simulink model "sfediticon"  (Simulink 7.6)
settings: Solver=FixedStepDiscrete  StartTime=0.0  StopTime=inf  RelTol=1e-3
CloseFcn:
  | sf_edit_icon('kill');
settings Model: Creator=The MathWorks Inc.  CovMetricSettings=dcmtr  ExtModeTrigMode=oneshot  ExtModeArmWhenConnect=off  ExtModeAutoUpdateStatusClock=off
settings DataIOCC: LimitDataPoints=off  SaveOutput=off  SaveTime=off
settings OptimizationCC: BooleanDataType=off  InlineInvariantSignals=on  InitFltsAndDblsToZero=on  EfficientMapNaN2IntZero=off
settings DebuggingCC: SaveWithParameterizedLinksMsg=none  SignalResolutionControl=TryResolveAllWithWarning  SolverPrmCheckMsg=none  MultiTaskDSMMsg=warning  MultiTaskCondExecSysMsg=none  StrictBusMsg=None
settings HardwareCC: TargetUnknown=on
settings SFSimCC: SimCustomHeaderCode=#define IS_MEX_TARGET 0  SimParseCustomCode=off
settings RTWCC: IncludeERTFirstTime=on
settings GRTTargetCC: TargetFcnLib=ansi_tfl_tmw.mat

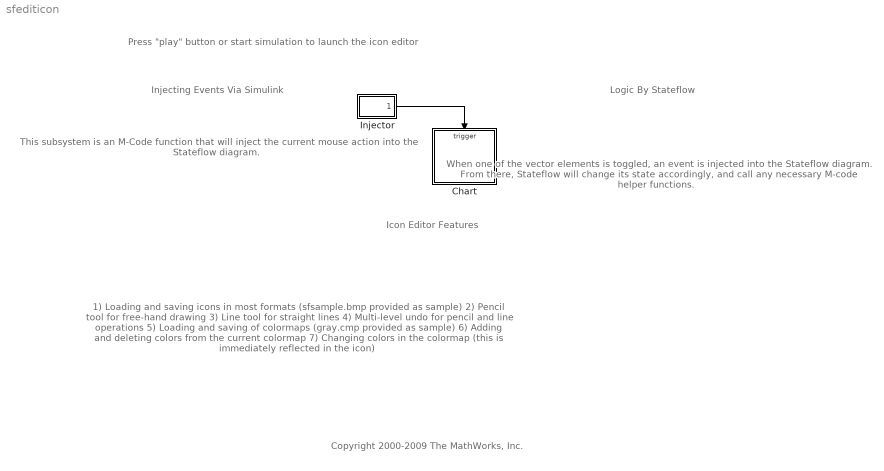
== system sfediticon ==
  note: This subsystem is an M-Code
      | function that will inject the
      | current mouse action into the
      | Stateflow diagram.
  note: Injecting Events
      | Via Simulink
  note: When one of the vector elements
      | is toggled, an event is injected
      | into the Stateflow diagram.
      | From there, Stateflow will
      | change its state accordingly,
      | and call any necessary M-code
      | helper functions.
  note: Logic By Stateflow
  note: 1) Loading and saving icons in most formats
      |      (sfsample.bmp provided as sample)
      | 2) Pencil tool for free-hand drawing
      | 3) Line tool for straight lines
      | 4) Multi-level undo for pencil and line operations
      | 5) Loading and saving of colormaps
      |      (gray.cmp provided as sample)
      | 6) Adding and deleting colors from the current
      |      colormap
      | 7) Changing colors in the colormap
      |     (this is immediately reflected in the icon)
  note: Icon Editor Features
  note: Press "play" button or start simulation to launch the icon editor
  note: Copyright 2000-2009 The MathWorks, Inc.
  Chart : Stateflow chart  TreatAsAtomicUnit=on
  Injector : Subsystem
  wires:
  Injector/1(Event) -> Chart/Trigger

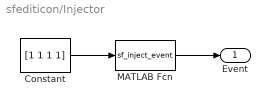
== system sfediticon/Injector ==
  Constant : Constant  Value=[1 1 1 1]
  MATLAB Fcn : MATLABFcn  MATLABFcn=sf_inject_event
  Event : Outport
  wires:
  MATLAB Fcn/1 -> Event/1
  Constant/1 -> MATLAB Fcn/1

== stateflow chart Chart ==
  settings: executeAtInitialization=1
  state ToolBar [parallel]
    settings: executionOrder=3
    state Released
    state Locked
      en:
      ml.sf_edit_icon...
      ('status', 'Tool locked');
    state Pressed
      en:
      pressedIcon = focusedIcon;
      press(pressedIcon,1);
      ex: press(pressedIcon,0);
    state icon_operation(icon) [function]
      (default) -> (junction 26)
      (junction 26) -> (junction 27) [order 2]
      (junction 26) -> (junction 28) [order 1] : [icon == OPEN_ICON] {ml.sf_edit_icon('open');}
      (junction 33) -> (junction 32) [order 1] : [icon == SAVE_MAP_ICON] {ml.sf_edit_icon('save_map');}
      (junction 27) -> (junction 29) [order 1] : [icon == SAVE_ICON] {ml.sf_edit_icon('save_as');}
      (junction 27) -> (junction 30) [order 2]
      (junction 30) -> (junction 31) [order 1] : [icon == OPEN_MAP_ICON] {ml.sf_edit_icon('open_map');}
      (junction 33) -> (junction 34) [order 2]
      (junction 34) -> (junction 70) : [icon == UNDO_ICON] {ml.sf_edit_icon('undo');}
      (junction 30) -> (junction 33) [order 2]
    state None
      pressedIcon = 0;
      ml.sf_edit_icon('status', 'Select a tool');
      ml.sf_edit_icon('normal_cursor');
    state press(icon,sp) [function]
      (junction 42) -> (junction 25) [order 2]
      (junction 35) -> (junction 37) [order 1] : [icon == OPEN_MAP_ICON] {ml.sf_edit_icon('press',sp,'open_map');}
      (junction 38) -> (junction 44) [order 1] : [icon == SAVE_MAP_ICON] {ml.sf_edit_icon('press', sp, 'save_map');}
      (junction 40) -> (junction 36) [order 1] : [icon == SAVE_ICON] {ml.sf_edit_icon('press', sp, 'save_as');}
      (junction 40) -> (junction 35) [order 2]
      (junction 35) -> (junction 38) [order 2]
      (junction 46) -> (junction 43) [order 1] : [icon == UNDO_ICON] {ml.sf_edit_icon('press',sp,'undo');}
      (junction 42) -> (junction 58) [order 1] : [icon == LINE_ICON] {ml.sf_edit_icon('press',sp,'line');}
      (junction 46) -> (junction 42) [order 2]
      (junction 38) -> (junction 46) [order 2]
      (junction 61) -> (junction 40) [order 2]
      (default) -> (junction 61)
      (junction 61) -> (junction 39) [order 1] : [icon == OPEN_ICON] {ml.sf_edit_icon('press', sp, 'open');}
      (junction 25) -> (junction 69) : [icon == PENCIL_ICON] {ml.sf_edit_icon('press',sp,'pencil');}
    ToolBar.None -> Pressed : NBD [in(Focus.Toolbar)]
    Released -> Pressed [order 1] : BM [pressedIcon == focusedIcon]
    Pressed -> Released [order 1] : BM [pressedIcon != focusedIcon]
    (junction 62) -> ToolBar.None [order 3] : {icon_operation(pressedIcon);}
    Released -> ToolBar.None [order 2] : BU
    (junction 62) -> Locked [order 1] : [(pressedIcon == LINE_ICON)]...
        | {ml.sf_edit_icon('line_cursor');}
    Locked -> Pressed : NBD[in(Focus.Toolbar)]
    (default) -> ToolBar.None
    (junction 62) -> Locked [order 2] : [(pressedIcon == PENCIL_ICON)]...
        | {ml.sf_edit_icon('pencil_cursor');}
    Pressed -> (junction 62) [order 2] : BU
  state Focus [parallel]
    settings: executionOrder=2
    state Palette
      state None
      state Swatch
      (junction 45) -> Focus.Palette.None [order 2]
      (junction 45) -> Swatch [order 1] : [ml.sf_edit_icon...
          | ('over_color_swatch')]
    state Icon
    state Canvas
    state None
    state Toolbar
      en: set_focusedIcon();
      du: set_focusedIcon();
      ex: focusedIcon = 0;
    state set_focusedIcon() [function]
      (default) -> (junction 48)
      (junction 48) -> (junction 49) [order 1] : [ml.sf_edit_icon('over_open_tool')] ...
          | {focusedIcon = OPEN_ICON;}
      (junction 48) -> (junction 50) [order 2]
      (junction 50) -> (junction 51) [order 1] : [ml.sf_edit_icon('over_saveas_tool')]...
          | {focusedIcon = SAVE_ICON;}
      (junction 50) -> (junction 52) [order 2]
      (junction 52) -> (junction 53) [order 1] : [ml.sf_edit_icon('over_openmap_tool')]...
          |  {focusedIcon = OPEN_MAP_ICON;}
      (junction 52) -> (junction 55) [order 2]
      (junction 55) -> (junction 54) [order 1] : [ml.sf_edit_icon('over_savemap_tool')] ...
          | {focusedIcon = SAVE_MAP_ICON;}
      (junction 55) -> (junction 56) [order 2]
      (junction 56) -> (junction 57) [order 1] : [ml.sf_edit_icon('over_undo_tool')]...
          |  {focusedIcon = UNDO_ICON;}
      (junction 65) -> (junction 47) [order 2] : {focusedIcon = 0;}
      (junction 56) -> (junction 63) [order 2]
      (junction 63) -> (junction 64) [order 1] : [ml.sf_edit_icon('over_line_tool')]...
          |  {focusedIcon = LINE_ICON;}
      (junction 63) -> (junction 65) [order 2]
      (junction 65) -> (junction 66) [order 1] : [ml.sf_edit_icon('over_pencil_tool')]...
          |  {focusedIcon = PENCIL_ICON;}
    (default) -> Focus.None
    (junction 41) -> Icon [order 4] : [ml.sf_edit_icon('over_icon')]
    (junction 41) -> Canvas [order 1] : [ml.sf_edit_icon('over_canvas')]
    (junction 41) -> Focus.None [order 5]
    Focus -> (junction 41) : BM
    (junction 41) -> (junction 45) [order 2] : [ml.sf_edit_icon('over_palette')]
    (junction 41) -> (junction 68) [order 3] : [ml.sf_edit_icon('over_toolbar')]
    (junction 68) -> Toolbar [order 2]
    (junction 68) -> (junction 59) [order 1] : [in(Toolbar)]
  state Main [parallel]
    settings: executionOrder=1
    state FGColorSelect
      en: ml.sf_edit_icon('cache_color');
      ex: ml.sf_edit_icon('fgcolor');
    state PencilDraw
      en: ml.sf_edit_icon('draw_point');
      du: ml.sf_edit_icon('draw_point');
      ex:  ml.sf_edit_icon('commit');
    state Idle
    state LineDraw
      en: ml.sf_edit_icon('anchor_line');
      du: ml.sf_edit_icon('render_line');
      ex:  ml.sf_edit_icon('commit');
    Idle -> (junction 67) [order 3] : ABD[in(Focus.Palette.Swatch)]
        | {ml.sf_edit_icon('show_color_menu');}
    Idle -> (junction 60) [order 1] : NBD[in(ToolBar.Locked)&&...
        |          in(Focus.Canvas)]
    Idle -> FGColorSelect [order 2] : NBD[in(Focus.Palette.Swatch)]
    (junction 60) -> PencilDraw [order 2] : [pressedIcon == PENCIL_ICON]
    (default) -> Idle : {ml.sf_edit_icon('create');}
    (junction 60) -> LineDraw [order 1] : [pressedIcon == LINE_ICON]
    Main -> Idle : BU
  state Note: [group]
    Make sure "Focus" comes before "Tool".
    The Tool state depends on up-to-date
    information about the Focus.
  data: icon function_input double; icon function_input double; sp function_input double; LINE_ICON constant int32 =1; OPEN_ICON constant int32 =2; OPEN_MAP_ICON constant int32 =3; PENCIL_ICON constant int32 =4; SAVE_MAP_ICON constant int32 =5; UNDO_ICON constant int32 =6; pressedIcon local int32; focusedIcon local int32; SAVE_ICON constant int32 =7
  events: BM input EITHER_EDGE_EVENT; NBD input EITHER_EDGE_EVENT; BU input EITHER_EDGE_EVENT; ABD input EITHER_EDGE_EVENT
